simulink model "TESA2Offense14"  (R2025b)
settings: Solver=FixedStepAuto  StartTime=0.0  StopTime=SimulationTime  FixedStep=timestep  RelTol=1e-3
values from neighbouring files (symbols this model uses):
  g = 9.81    [TESA_Workspace1.m]    (also in TESA_Workspace2.m)
  I = eye(3,3)    [TESA_Workspace1.m]    (also in TESA_Workspace2.m)
  K = [1 1 1 1 ... (first row only)    [TESA_Workspace1.m]    (also in TESA_Workspace2.m)
  Kp = 1*Kp    [TESA_Workspace2.m]
  Kr = 1*Kr    [TESA_Workspace2.m]
  Kv = 1*Kv    [TESA_Workspace2.m]
  Kw = 1*Kw    [TESA_Workspace2.m]
  m = 4.34    [TESA_Workspace1.m]    (also in TESA_Workspace2.m)
undefined symbols (not defined in the file or in its folder): alt_init, fense_lats, fense_lons, fractalcoef, lat_init, long_init, reai, test
libraries: mqttlib x1, sensorgpslib x1, mspsensorlib x1
settings Model: Creator=worap  LastModifiedBy=IXVIA
settings DataIOCC: ExternalInput=inputStructure  LoadExternalInput=on
settings ConfigSetCC: MQTTTableInfo=[]

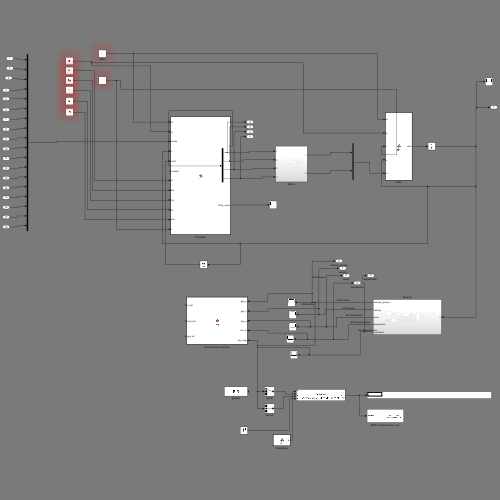
[thumbnail: Simulink's stored preview of the top-level diagram]
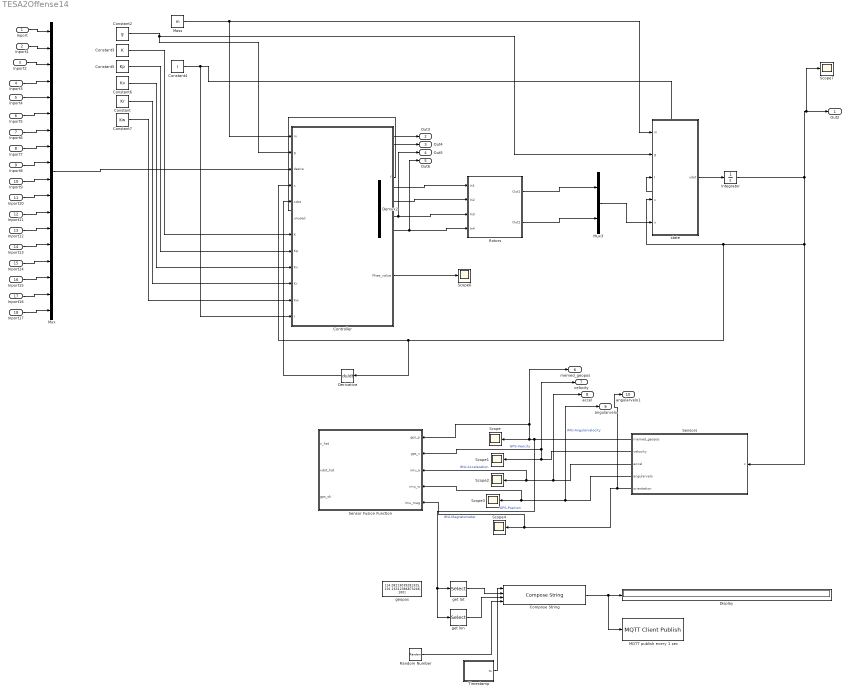
== system TESA2Offense14 ==
  Inport : Inport
  Inport1 : Inport  Port=2
  Inport2 : Inport  Port=3
  Inport3 : Inport  Port=4
  Inport4 : Inport  Port=5
  Inport5 : Inport  Port=6
  Inport6 : Inport  Port=7
  Inport7 : Inport  Port=8
  Inport8 : Inport  Port=9
  Inport9 : Inport  Port=10
  Inport10 : Inport  Port=11
  Inport11 : Inport  Port=12
  Inport12 : Inport  Port=13
  Inport13 : Inport  Port=14
  Inport14 : Inport  Port=15
  Inport15 : Inport  Port=16
  Inport16 : Inport  Port=17
  Inport17 : Inport  Port=18
  Compose String : ComposeString  Format="'{ \\\"timestamp \\\": %f, \\\"latitude \\\": %f, \\\"longitude\\\": %f, \\\"altitude \\\": %f }'"
  Constant : Constant  Value=Kr
  Constant2 : Constant  Value=g
  Constant3 : Constant  Value=K
  Constant4 : Constant  Value=I
  Constant5 : Constant  Value=Kp
  Constant6 : Constant  Value=Kv
  Constant7 : Constant  Value=Kw
  Controller : MATLAB Function  TreatAsAtomicUnit=on
  Demux2 : Demux
  Derivative : Derivative
  Display : Display
  Integrator : Integrator  InitialCondition=[0;0;0;0;0;0;1;0;0;0;1;0;0;0;1;0;0;0]
  MQTT publish every 1 sec : mqttlib/MQTT Client Publish  RetainClient=MQTTClient  ClientList=MQTTClient  TopicsTable={ '1', 'reai/test', '0', 'false' }  PublishOnDataChange=off  SampleTime=1  TopicNames=reai/test  NumTopics=1  IsLib=0  BlkName=MQTT Client Publish
  Mass : Constant  Value=m
  Mux : Mux  Inputs=18
  Mux3 : Mux  Inputs=2
  Random Number : RandomNumber  SampleTime=1
  Rotors : Subsystem
  Scope{,1..4,6..7} (7 alike) : Scope
      Scope settings: ActiveDisplayYMinimum=-392.49114665190103  ActiveDisplayYMaximum=418.7762343955248
      Scope1 settings: ActiveDisplayYMinimum=-3502.8833679211148  ActiveDisplayYMaximum=3575.603681327907  DataLoggingVariableName=ScopeData2
      Scope2 settings: ActiveDisplayYMinimum=-1798.8130288406041  ActiveDisplayYMaximum=1151.8108947334445  DataLoggingVariableName=ScopeData3
      Scope3 settings: ActiveDisplayYMinimum=-57.363961461922528  ActiveDisplayYMaximum=117.62406798675227  DataLoggingVariableName=ScopeData4
      Scope4 settings: ActiveDisplayYMinimum=-40.166345129221554  ActiveDisplayYMaximum=42.415838093401533  DataLoggingVariableName=ScopeData5
      Scope6 settings: ActiveDisplayYMinimum=-0.10349  ActiveDisplayYMaximum=2.21622
      Scope7 settings: ActiveDisplayYMinimum=-13370.290018848573  ActiveDisplayYMaximum=18920.015749277885  DataLoggingVariableName=ScopeData7
  Sensor Fusion Function : MATLAB Function  TreatAsAtomicUnit=on
  Sensors : Subsystem
  Timestamp : MATLAB Function  TreatAsAtomicUnit=on
  geopos : Constant  Value=[14.28213039281325, 101.16312386873248, 100]
  get lat : Selector  InputPortWidth=3  IndexOptions=Index vector (dialog)  Indices=[1]  OutputSizes=1
  get lon : Selector  InputPortWidth=3  IndexOptions=Index vector (dialog)  Indices=[2]  OutputSizes=1
  state : MATLAB Function  TreatAsAtomicUnit=on
  Out2 : Outport
  Out3 : Outport  Port=2
  Out4 : Outport  Port=3
  Out5 : Outport  Port=4
  Out6 : Outport  Port=5
  memed_geopos : Outport  Port=6
  velocity : Outport  Port=7
  accel : Outport  Port=8
  angularvelo : Outport  Port=9
  angularvelo1 : Outport  Port=10
  wires:
  Mass/1 -> state/1(m), Controller/1(m)
  Demux2/2 -> Out4/1, Rotors/2(In2)
  Rotors/1(Out1) -> Mux3/1
  Rotors/2(Out2) -> Mux3/2
  Demux2/3 -> Out5/1, Rotors/3(In3)
  Demux2/4 -> Out6/1, Rotors/4(In4)
  Controller/1(f) -> Demux2/1
  Demux2/1 -> Out3/1, Rotors/1(In1)
  Constant2/1 -> state/2(g), Controller/2(g)
  Constant3/1 -> Controller/7(K)
  Constant5/1 -> Controller/8(Kp)
  Constant6/1 -> Controller/9(Kv)
  Constant7/1 -> Controller/11(Kw)
  Constant/1 -> Controller/10(Kr)
  Controller/2(Phee_value) -> Scope6/1
  Mux3/1 -> state/5(u)
  Integrator/1 -> Scope7/1, Out2/1, Sensors/1(x), Derivative/1, Controller/4(x), state/4(x)
  Mux/1 -> Controller/3(desire)
  Inport17/1 -> Mux/18
  Inport16/1 -> Mux/17
  Inport15/1 -> Mux/16
  Inport14/1 -> Mux/15
  Inport13/1 -> Mux/14
  Inport12/1 -> Mux/13
  Inport11/1 -> Mux/12
  Inport10/1 -> Mux/11
  Inport9/1 -> Mux/10
  Inport8/1 -> Mux/9
  Inport7/1 -> Mux/8
  Inport6/1 -> Mux/7
  Inport5/1 -> Mux/6
  Inport4/1 -> Mux/5
  Inport3/1 -> Mux/4
  Inport2/1 -> Mux/3
  Inport1/1 -> Mux/2
  Inport/1 -> Mux/1
  Sensors/1(memed_geopos) -> get lon/1, get lat/1, Scope/1, Sensor Fusion Function/1(gps_p), memed_geopos/1  "GPS-Position"
  Sensors/2(velocity) -> Sensor Fusion Function/2(gps_v), velocity/1, Scope1/1  "GPS-Veocity"
  Sensors/3(accel) -> accel/1, Sensor Fusion Function/3(imu_a), Scope2/1  "IMU-Accelaration"
  Sensors/4(angularvelo) -> angularvelo/1, Sensor Fusion Function/4(imu_w), Scope3/1  "IMU-Angularvelocity"
  Sensors/5(orientation) -> angularvelo1/1, Sensor Fusion Function/5(imu_mag), Scope4/1  "IMU-Magnetometer"
  Constant4/1 -> Controller/12(I), state/3(I)
  state/1(xdot) -> Integrator/1
  get lat/1 -> Compose String/2
  Compose String/1 -> MQTT publish every 1 sec/1, Display/1
  Random Number/1 -> Compose String/4
  Timestamp/1(ts) -> Compose String/1
  get lon/1 -> Compose String/3
  Derivative/1 -> Controller/5(xdot)

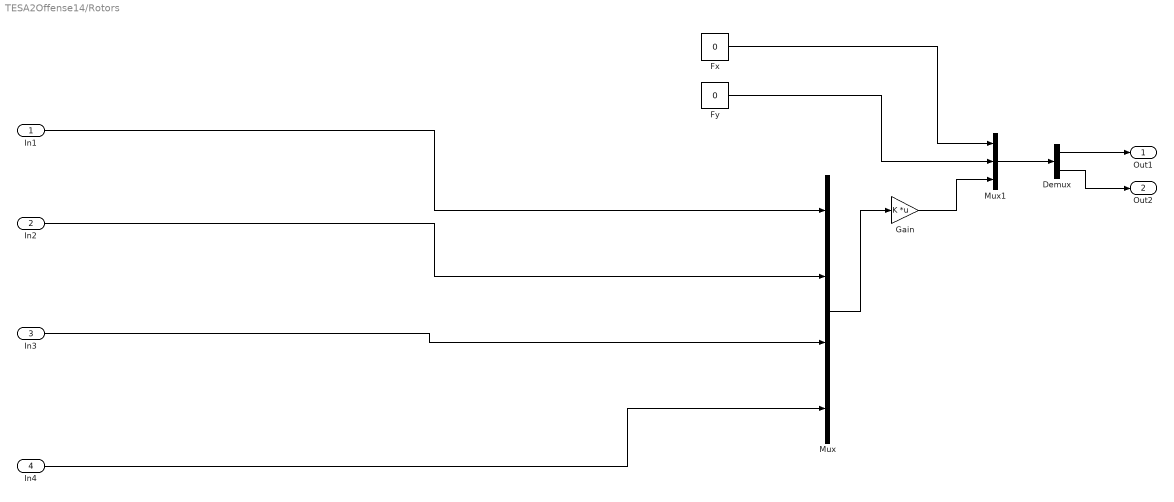
== system TESA2Offense14/Rotors ==
  In1 : Inport
  In2 : Inport  Port=2
  In3 : Inport  Port=3
  In4 : Inport  Port=4
  Demux : Demux  Outputs=2
  Fx : Constant  Value=0
  Fy : Constant  Value=0
  Gain : Gain  Gain=K  Multiplication=Matrix(K*u) (u vector)
  Mux : Mux
  Mux1 : Mux  Inputs=3
  Out1 : Outport
  Out2 : Outport  Port=2
  wires:
  Fx/1 -> Mux1/1
  Mux1/1 -> Demux/1
  Fy/1 -> Mux1/2
  Mux/1 -> Gain/1
  Gain/1 -> Mux1/3
  Demux/2 -> Out2/1
  Demux/1 -> Out1/1
  In1/1 -> Mux/1
  In2/1 -> Mux/2
  In3/1 -> Mux/3
  In4/1 -> Mux/4

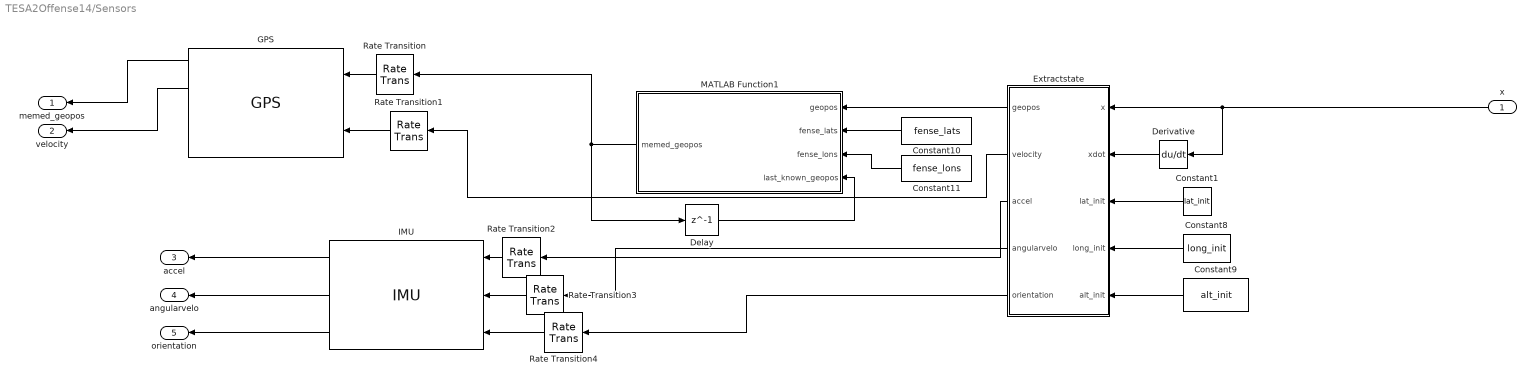
== system TESA2Offense14/Sensors ==
  x : Inport
  Constant1 : Constant  Value=lat_init
  Constant10 : Constant  Value=fense_lats
  Constant11 : Constant  Value=fense_lons
  Constant8 : Constant  Value=long_init
  Constant9 : Constant  Value=alt_init
  Delay : Delay  DelayLength=1  InitialCondition=0
  Derivative : Derivative
  Extractstate : MATLAB Function  TreatAsAtomicUnit=on
  GPS : sensorgpslib/GPS  DispRefFrame=NED  PositionInputFormat=Geodetic  ReferenceLocation=[ 0, 0, 0 ]  HorizontalPositionAccuracy=1.6  VerticalPositionAccuracy=3  VelocityAccuracy=0.1  DecayFactor=0.999  SeedDouble=67  SimulateUsing=Interpreted execution
      settings: LibrarySourceBlock=mspsensorlib/GPS
  IMU : mspsensorlib/IMU  DispRefFrame=NED  TemperaturePort=off  Temperature=25  MagneticFieldPort=off  MagneticFieldNED=[ 27.5550, -2.4169, -16.0849 ]  MagneticFieldENU=[ -2.4169, 27.5550, 16.0849 ]  SeedDouble=67  SimulateUsing=Interpreted execution  AccelParamsMeasurementRange=Inf  AccelParamsResolution=0  AccelParamsConstantBias=[ 0, 0, 0 ]  AccelParamsAxesMisalignment=[ 100, 0, 0; 0, 100, 0; 0, 0, 100 ]  AccelParamsNoiseDensity=[ 0.003924 0.003924 0.003924 ]  AccelParamsBiasInstability=[ 0, 0, 0 ]  AccelParamsBiasInstabilityNumerator=fractalcoef().Numerator  AccelParamsBiasInstabilityDenominator=fractalcoef().Denominator  AccelParamsRandomWalk=[ 0, 0, 0 ]  AccelParamsNoiseType=double-sided  AccelParamsTemperatureBias=[ 0, 0, 0 ]  AccelParamsTemperatureScaleFactor=[ 0, 0, 0 ]  GyroParamsMeasurementRange=Inf  GyroParamsResolution=0  GyroParamsConstantBias=[ 0, 0, 0 ]  GyroParamsAxesMisalignment=[ 100, 0, 0; 0, 100, 0; 0, 0, 100 ]  GyroParamsAccelerationBias=[ 0, 0, 0 ]  GyroParamsNoiseDensity=[ 0.0125, 0.0125, 0.0125 ]  GyroParamsBiasInstability=[ 0, 0, 0 ]  GyroParamsBiasInstabilityNumerator=fractalcoef().Numerator  GyroParamsBiasInstabilityDenominator=fractalcoef().Denominator  GyroParamsRandomWalk=[ 0, 0, 0 ]  GyroParamsNoiseType=double-sided  GyroParamsTemperatureBias=[ 0, 0, 0 ]  GyroParamsTemperatureScaleFactor=[ 0, 0, 0 ]  MagParamsMeasurementRange=Inf  MagParamsResolution=0  MagParamsConstantBias=[ 0, 0, 0 ]  MagParamsAxesMisalignment=[ 100, 0, 0; 0, 100, 0; 0, 0, 100 ]  MagParamsNoiseDensity=[0.6 0.6 0.9]/sqrt(100)  MagParamsBiasInstability=[ 0, 0, 0 ]  MagParamsBiasInstabilityNumerator=fractalcoef().Numerator  MagParamsBiasInstabilityDenominator=fractalcoef().Denominator  MagParamsRandomWalk=[ 0, 0, 0 ]  MagParamsNoiseType=double-sided  MagParamsTemperatureBias=[ 0, 0, 0 ]  MagParamsTemperatureScaleFactor=[ 0, 0, 0 ]
  MATLAB Function1 : MATLAB Function  TreatAsAtomicUnit=on
  Rate Transition{,1..4} (5 alike) : RateTransition
  memed_geopos : Outport
  velocity : Outport  Port=2
  accel : Outport  Port=3
  angularvelo : Outport  Port=4
  orientation : Outport  Port=5
  wires:
  Constant11/1 -> MATLAB Function1/3(fense_lons)
  Constant8/1 -> Extractstate/4(long_init)
  Constant1/1 -> Extractstate/3(lat_init)
  Constant10/1 -> MATLAB Function1/2(fense_lats)
  Delay/1 -> MATLAB Function1/4(last_known_geopos)
  Derivative/1 -> Extractstate/2(xdot)
  Constant9/1 -> Extractstate/5(alt_init)
  Extractstate/1(geopos) -> MATLAB Function1/1(geopos)
  MATLAB Function1/1(memed_geopos) -> Delay/1, Rate Transition/1
  x/1 -> Derivative/1, Extractstate/1(x)
  IMU/1 -> accel/1
  IMU/2 -> angularvelo/1
  IMU/3 -> orientation/1
  Extractstate/3(accel) -> Rate Transition2/1
  Extractstate/4(angularvelo) -> Rate Transition3/1
  Extractstate/5(orientation) -> Rate Transition4/1
  Extractstate/2(velocity) -> Rate Transition1/1
  GPS/1 -> memed_geopos/1
  GPS/2 -> velocity/1
  Rate Transition/1 -> GPS/1
  Rate Transition1/1 -> GPS/2
  Rate Transition2/1 -> IMU/1
  Rate Transition3/1 -> IMU/2
  Rate Transition4/1 -> IMU/3

== matlab function TESA2Offense14/Timestamp ==
  data: ts output
function ts = fcn()
    % Real-world UNIX timestamp
    ts = posixtime(datetime('now'));
end

== matlab function TESA2Offense14/state ==
  data: m input; g input; I input; x input; u input; xdot output
function xdot = fcn(m,g,I,x,u)

% extract the x-vextor
p = x(1:3,1);
v = x(4:6,1);
R = reshape(x(7:15,1),3,3);
omega = x(16:18,1);

%control signal
f = u(3,1);
M = u(4:6,1);

e3 = [0;0;1];


xdot = zeros(size(x));

xdot(1:3,1) = v;
xdot(4:6,1) = g*e3 - 1/m*f*R*e3;

Rdot = R*hatmap(omega);
xdot(7:15,1) = Rdot(:);

xdot(16:18,1) = I\(M - cross(omega,I*omega));




end

== matlab function TESA2Offense14/Controller ==
  data: m input; g input; f output; Phee_value output; desire input; x input; xdot input; unused input; K input; Kp input; Kv input; Kr input; Kw input; I input
function [f, Phee_value] = fcn(m, g, desire, x, xdot, ~, K, Kp, Kv, Kr, Kw, I)
%#codegen

% ---- preallocate outputs (fix dims) ----
f = zeros(4,1);
Phee_value = 0;

e3 = [0;0;1];


% -------- desired --------
rd    = desire(1:3);
vd    = desire(4:6);
ad    = desire(7:9);
jd    = desire(10:12);    
psid  = desire(16);
dpsid = desire(17);

% -------- actual --------
p = x(1:3);
v = x(4:6);          % เดิมใช้ xdot → ผิดแน่นอน
R = reshape(x(7:15),3,3);
omega = x(16:18);

phi = atan2(R(3,2), R(3,3));
Phee_value = phi;

% -------- gains --------
if isempty(I), I = eye(3); end
Ix = I(1,1); Iy = I(2,2); Iz = I(3,3);

Kp = diag([4.0*m, 4.0*m, 12.0*m]);
Kv = diag([8.0*m, 8.0*m, 10.0*m]);
Kr = diag([(8.0^2)*Ix, (8.0^2)*Iy, (5.5^2)*Iz]);
Kw = diag([2*8.0*Ix,   2*8.0*Iy,   2*5.5*Iz]);

% -------- force with feedforward --------
dt = 0.01;                       % ให้ตรงกับ sample time ของบล็อก
jerk_ff = 0;

vel_error_magnitude = norm(v - vd);
vel_ff_gain = min(0.25, norm(v - vd) / 4.0);
vel_ff = vel_ff_gain * m * (ad - [0;0;g]);

A = -Kp*(p-rd) - Kv*(v-vd) - m*g*e3 + m*ad + jerk_ff + vel_ff;

A_norm = norm(A);
if A_norm < 1e-9
    A = -m*g*e3; A_norm = m*g;
end

% -------- desired attitude --------
b3c = -A / A_norm;
cpsi = cos(psid); spsi = sin(psid);
b1d  = [cpsi; spsi; 0];
b2c  = cross(b3c,b1d); nb2 = norm(b2c);
if nb2 < 1e-9
    b1d=[cpsi;spsi;1e-3]; b2c=cross(b3c,b1d); nb2=norm(b2c);
    if nb2 < 1e-12, nb2 = 1e-12; end
end
b2c = b2c/nb2;  b1c = cross(b2c,b3c);
Rc  = [b1c,b2c,b3c];

% -------- attitude errors --------
eR_mat = 0.5*(Rc.'*R - R.'*Rc);
eR = [eR_mat(3,2); eR_mat(1,3); eR_mat(2,1)];
eOmega = omega - (R.'*Rc)*[0;0;dpsid];

% -------- thrust & moments --------
Re3 = R*e3;
T = -A.'*Re3;
M = -Kr*eR - Kw*eOmega;

% thrust & moment limits
if ~isfinite(T), T = m*g; end
T = max(0.05*m*g, min(T, 3.5*m*g));

M_max = [1.0; 1.0; 0.4];
for i=1:3
    if ~isfinite(M(i)), M(i)=0; end
    M(i) = max(-M_max(i), min(M(i), M_max(i)));
end

% -------- allocation --------
U = [T; M];
omega2 = K \ U;
f = omega2;

end

== matlab function TESA2Offense14/Sensors/Extractstate ==
  data: geopos output; velocity output; x input; accel output; xdot input; angularvelo output; orientation output; lat_init input; long_init input; alt_init input
function [geopos, velocity,accel, angularvelo, orientation] = Extractstate(x,xdot,lat_init,long_init,alt_init)

position = x(1:3)';
velocity = x(4:6)';
accel = xdot(4:6)';
R = x(7:15);
orientation = reshape(R,3,3);
angularvelo = x(16:18)';


geopos = ned2lla(position, [lat_init long_init alt_init], "ellipsoid");

end

== matlab function TESA2Offense14/Sensors/MATLAB Function1 ==
  data: geopos input; memed_geopos output; fense_lats input; fense_lons input; last_known_geopos input
function memed_geopos  = is_jammed(geopos, fense_lats, fense_lons, last_known_geopos)
    
    memed_geopos = geopos;

    if fense_lats ~= 0
        if (geopos(1) > min(fense_lats)) && (geopos(1) < max(fense_lats)) && (geopos(2) > min(fense_lons)) && (geopos(2) < max(fense_lons))
            memed_geopos = [14.30613815134626, 101.18904132968885, 30];
        end
    end
end

== matlab function TESA2Offense14/Sensor Fusion Function ==
  data: gps_p input; x_hat output double size=[18 1]; gps_v input; imu_a input; imu_w input; imu_mag input; xdot_hat output size=[18 1]; gps_ok output size=1
function [x_hat, xdot_hat, gps_ok] = fcn(gps_p, gps_v, imu_a, imu_w, imu_mag)
%#codegen
% Discrete Sensor Fusion (Complementary + anti-spoof) for quadrotor (NED)
% Outputs:
%   x_hat(18x1)  = [p(1:3); v(4:6); vec(Rb2n)(7:15); omega(16:18)]
%   xdot_hat(18x1)= [pdot; vdot; vec(Rdot)(7:15); omegadot]
%   gps_ok       = true when GPS trusted (not spoof/hold)

% ---------- enforce column 3x1 ----------
gps_p   = reshape(gps_p,  3,1);
gps_v   = reshape(gps_v,  3,1);
imu_a   = reshape(imu_a,  3,1);
imu_w   = reshape(imu_w,  3,1);
imu_mag = reshape(imu_mag,3,1);

% ---------- outputs fixed-size ----------
x_hat     = coder.nullcopy(zeros(18,1));
xdot_hat  = coder.nullcopy(zeros(18,1));
gps_ok    = false;

% ---------- params ----------
Ts         = 0.01;     % sample [s]
g          = 9.81;
alpha_p    = 0.12;     % GPS blend pos
alpha_v    = 0.18;     % GPS blend vel
Kacc       = 0.02;     % tilt fix from acc
Kmag       = 0.02;     % yaw fix from mag
jump_thr_m = 8.0;      % GPS jump [m]
innov_thr  = 30.0;     % innovation [m]
hold_N     = int32(200);   % steps to hold IMU-only
betaOmega  = 0.3;      % LPF for omega (0..1)
% anti-burst (จำกัดความชันเมื่อกลับไปใช้ GPS)
max_dp_per_step = 2.0; % m/step
max_dv_per_step = 3.0; % m/s per step

% ---------- persistent ----------
persistent p_hat v_hat Rb2n last_gps spoof_cnt omega_hat init_done
if isempty(init_done)
    p_hat = zeros(3,1);
    v_hat = zeros(3,1);
    Rb2n  = eye(3);
    last_gps  = gps_p;
    spoof_cnt = int32(0);
    omega_hat = zeros(3,1);
    init_done = true;
end

% ===== 1) Attitude update (gyro + acc tilt + mag yaw) =====
% 1.1 integrate gyro (small-angle)
dth  = imu_w * Ts;
Rb2n = Rb2n * (eye(3)+skew(dth));
Rb2n = orthonormalize(Rb2n);

% 1.2 tilt correction using accelerometer (align gravity)
gb_est_b = Rb2n' * [0;0;g];
na = norm(imu_a); ngb = norm(gb_est_b);
if (na > 1e-9) && (ngb > 1e-9)
    e_tilt = cross( imu_a/na, gb_est_b/ngb );
    Rb2n   = Rb2n * (eye(3)+skew(-Kacc*e_tilt));
    Rb2n   = orthonormalize(Rb2n);
end

% 1.3 yaw correction using magnetometer
nm = norm(imu_mag);
if nm > 1e-9
    mn       = Rb2n * (imu_mag/nm);
    yaw_meas = atan2(mn(2), mn(1));
    yaw_est  = atan2(Rb2n(2,1), Rb2n(1,1));
    dyaw     = wrapToPi(yaw_meas - yaw_est);
    Rb2n     = rotZ(Kmag*dyaw) * Rb2n;
    Rb2n     = orthonormalize(Rb2n);
end

% ===== 2) Predict (IMU-only) =====
% specific force to NED (a_n = Rb2n*a_b + g)
a_n   = Rb2n*imu_a + [0;0;g];
v_prd = v_hat + a_n*Ts;
p_prd = p_hat + v_prd*Ts;

% ===== 3) Spoof detection =====
jump  = norm(gps_p - last_gps);
innov = norm(gps_p - p_prd);
use_gps = true;
if (jump > jump_thr_m) || (innov > innov_thr) || (spoof_cnt > 0)
    use_gps = false;
end
if (jump > jump_thr_m) || (innov > innov_thr)
    spoof_cnt = hold_N;
elseif spoof_cnt > 0
    spoof_cnt = spoof_cnt - 1;
end
last_gps = gps_p;
gps_ok = use_gps;

% ===== 4) Update =====
if use_gps
    % blend + anti-burst limiter
    p_cand = (1-alpha_p)*p_prd + alpha_p*gps_p;
    v_cand = (1-alpha_v)*v_prd + alpha_v*gps_v;

    dp = p_cand - p_hat;
    dv = v_cand - v_hat;
    lim = max_dp_per_step/max(1e-9,norm(dp));
    if lim < 1.0, dp = dp*lim; end
    limv = max_dv_per_step/max(1e-9,norm(dv));
    if limv < 1.0, dv = dv*limv; end

    p_hat = p_hat + dp;
    v_hat = v_hat + dv;
else
    p_hat = p_prd;
    v_hat = v_prd;
end

% ===== 5) Omega estimate (LPF) =====
omega_hat = (1-betaOmega)*omega_hat + betaOmega*imu_w;

% ===== 6) Pack x_hat (18x1) =====
x_hat(1:3)  = p_hat;
x_hat(4:6)  = v_hat;
x_hat(7:15) = [Rb2n(1,1);Rb2n(2,1);Rb2n(3,1); Rb2n(1,2);Rb2n(2,2);Rb2n(3,2); Rb2n(1,3);Rb2n(2,3);Rb2n(3,3)];
x_hat(16:18)= omega_hat;

% ===== 7) Build xdot_hat (18x1) =====
% ṗ = v;  v̇ = a_n;  Ṙ = R·skew(ω̂);  ω̇ ~ LPF derivative (หรือศูนย์)
x_dot_p = v_hat;
x_dot_v = a_n;
Rdot    = Rb2n*skew(omega_hat);
x_dot_R = [Rdot(1,1);Rdot(2,1);Rdot(3,1); Rdot(1,2);Rdot(2,2);Rdot(3,2); Rdot(1,3);Rdot(2,3);Rdot(3,3)];
x_dot_w = (omega_hat - imu_w)*0; % ใช้ 0 เพื่อไม่ใส่อนุพันธ์รบกวน (จะใส่ฟิลเตอร์ภายนอกก็ได้)

xdot_hat(1:3)   = x_dot_p;
xdot_hat(4:6)   = x_dot_v;
xdot_hat(7:15)  = x_dot_R;
xdot_hat(16:18) = x_dot_w;

% ===== helpers =====
function S = skew(w)
S = zeros(3,3);
S(1,2)=-w(3); S(1,3)= w(2);
S(2,1)= w(3); S(2,3)=-w(1);
S(3,1)=-w(2); S(3,2)= w(1);
end
function Rn = orthonormalize(R)
% fast Gram-Schmidt
x = R(:,1); x = x / max(1e-12, norm(x));
y = R(:,2) - x*(x.'*R(:,2)); y = y / max(1e-12, norm(y));
z = [ x(2)*y(3)-x(3)*y(2);
      x(3)*y(1)-x(1)*y(3);
      x(1)*y(2)-x(2)*y(1) ];
% right-handed
if x(1)*(y(2)*z(3)-y(3)*z(2)) - x(2)*(y(1)*z(3)-y(3)*z(1)) + x(3)*(y(1)*z(2)-y(2)*z(1)) < 0
    z = -z;
end
Rn = [x y z];
end
function a = wrapToPi(a)
a = mod(a+pi, 2*pi) - pi;
end
function Rz = rotZ(a)
ca = cos(a); sa = sin(a);
Rz = [ca -sa 0; sa ca 0; 0 0 1];
end
end
